simulink model "mfbDouble"  (R2020b)
settings: Solver=VariableStepAuto  StartTime=0.0  StopTime=10.0  RelTol=1e-3
settings Model: Creator=Rocksmithed  LastModifiedBy=Rocksmithed

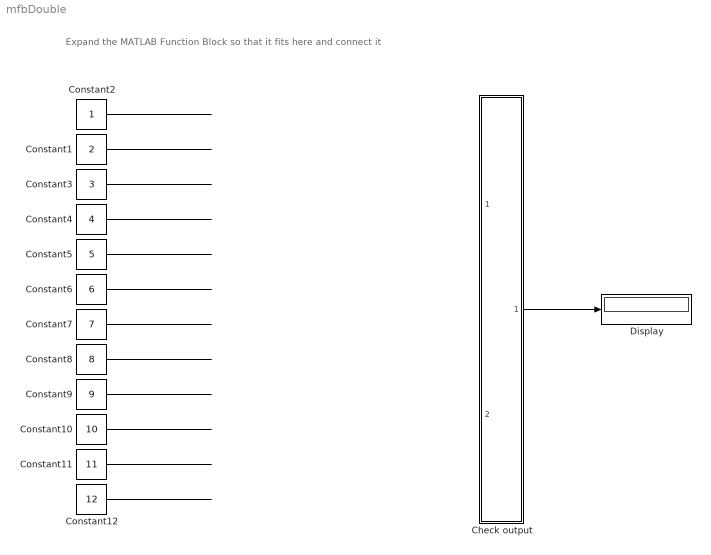
== system mfbDouble ==
  note: Expand the MATLAB Function Block so that it fits here and connect it
  Check output : Subsystem
  Constant1 : Constant  Value=2
  Constant10 : Constant  Value=10
  Constant11 : Constant  Value=11
  Constant12 : Constant  Value=12
  Constant2 : Constant
  Constant3 : Constant  Value=3
  Constant4 : Constant  Value=4
  Constant5 : Constant  Value=5
  Constant6 : Constant  Value=6
  Constant7 : Constant  Value=7
  Constant8 : Constant  Value=8
  Constant9 : Constant  Value=9
  Display : Display
  wires:
  Constant2/1 -> ?
  Constant1/1 -> ?
  Constant3/1 -> ?
  Constant4/1 -> ?
  Constant5/1 -> ?
  Constant6/1 -> ?
  Constant7/1 -> ?
  Constant8/1 -> ?
  Constant9/1 -> ?
  Constant10/1 -> ?
  Constant11/1 -> ?
  Constant12/1 -> ?
  ? -> Check output/2(xddot2)
  Check output/1(Out1) -> Display/1
  ? -> Check output/1(xddot1)

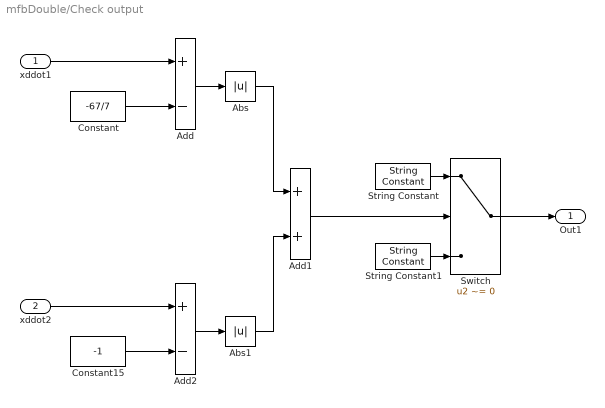
== system mfbDouble/Check output ==
  xddot1 : Inport
  xddot2 : Inport  Port=2
  Abs : Abs
  Abs1 : Abs
  Add : Sum  Inputs=+-
  Add1 : Sum
  Add2 : Sum  Inputs=+-
  Constant : Constant  Value=-67/7
  Constant15 : Constant  Value=-1
  String Constant : StringConstant  String="\"Incorrect\""
  String Constant1 : StringConstant  String="\"Correct\""
  Switch : Switch  Criteria=u2 ~= 0
  Out1 : Outport
  wires:
  Constant15/1 -> Add2/2
  Constant/1 -> Add/2
  String Constant1/1 -> Switch/3
  Abs/1 -> Add1/1
  Add2/1 -> Abs1/1
  Abs1/1 -> Add1/2
  Add/1 -> Abs/1
  xddot2/1 -> Add2/1
  String Constant/1 -> Switch/1
  xddot1/1 -> Add/1
  Switch/1 -> Out1/1
  Add1/1 -> Switch/2
